simulink model "test_Cart_ver6"  (R2018a)
settings: Solver=VariableStepAuto  StartTime=0.0  StopTime=inf  RelTol=1e-3
undefined symbols (not defined in the file): first, serial, termDistance
libraries: instrumentlib x3, sldrtlib x1, simulink x1
settings Model: Creator=tomato  LastModifiedBy=tomatoPC
settings CodeAppCC: StateflowObjectComments=on

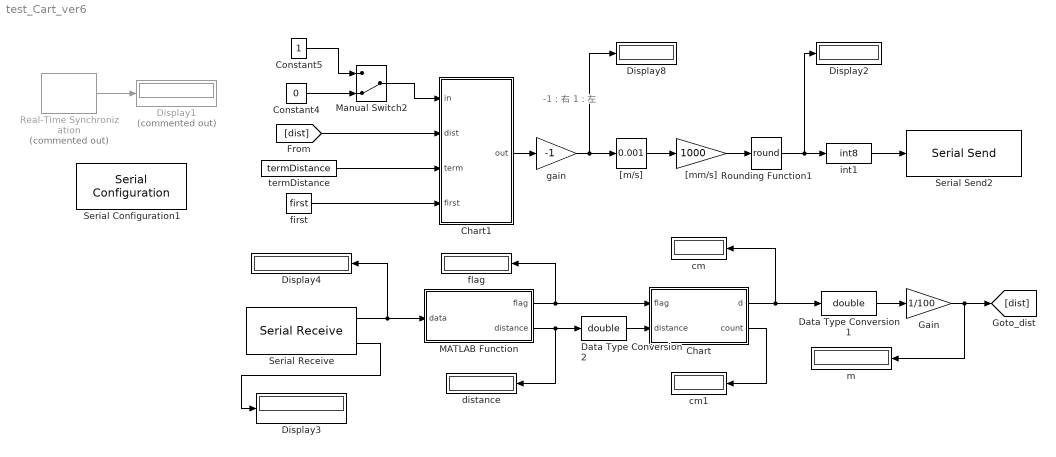
== system test_Cart_ver6 ==
  note: -1 : 右
      | 1 : 左
  Chart : Stateflow chart  TreatAsAtomicUnit=on
  Chart1 : Stateflow chart  TreatAsAtomicUnit=on
  Constant4 : Constant  Value=0  SampleTime=1
  Constant5 : Constant  SampleTime=1
  Data Type Conversion1 : DataTypeConversion  OutDataTypeStr=double
  Data Type Conversion2 : DataTypeConversion  OutDataTypeStr=double
  Display1 : Display  Commented=on
  Display{2..4,8} (4 alike) : Display
  Gain : Gain  Gain=1/100
  MATLAB Function : MATLAB Function  TreatAsAtomicUnit=on
  Manual Switch2 : ManualSwitch  CurrentSetting=0
  Real-Time Synchronization : sldrtlib/Real-Time Synchronization  Commented=on  SampleTime=1  MaxMissedTicks=inf  ShowMissedTicks=on  YieldWhenWaiting=off
  Rounding Function1 : Rounding  Operator=round
  Serial Configuration1 : instrumentlib/Serial Configuration  Priority=-200000  ComPortMenu=<Please select a port...>  ComPort=COM8  ObjConstructor=serial('COM8');  BaudRate=115200  DataBits=8  Parity=none  StopBits=1  FlowControl=none  Timeout=10  ByteOrder=LittleEndian
  Serial Receive : instrumentlib/Serial Receive  ComPortMenu=<Please select a port...>  ComPort=COM8  ObjConstructor=serial('COM8');  Terminator=<none>  DataSize=1  DataType=uint8  EnableBlockingMode=off  ActionDataUnavailable=Output last received value  CustomValue=0  SampleTime=0.01
  Serial Send2 : instrumentlib/Serial Send  ComPortMenu=<Please select a port...>  ComPort=COM8  ObjConstructor=serial('COM8');  Terminator=<none>  EnableBlockingMode=on
  "[m/s]" : simulink/Math Operations/Slider Gain  gain=0.001  low=-0.128  high=0.127
  "[mm/s]" : Gain  Gain=1000
  cm : Display
  cm1 : Display
  distance : Display
  first : Constant  Value=first  SampleTime=1
  flag : Display
  gain : Gain  Gain=-1
  int1 : DataTypeConversion  OutDataTypeStr=int8
  m : Display
  termDistance : Constant  Value=termDistance  SampleTime=1
  wires:
  gain/1 -> "[m/s]"/1, Display8/1
  "[m/s]"/1 -> "[mm/s]"/1
  int1/1 -> Serial Send2/1
  Serial Receive/2 -> Display3/1
  Chart1/1(out) -> gain/1
  "[mm/s]"/1 -> Rounding Function1/1
  termDistance/1 -> Chart1/3(term)
  Manual Switch2/1 -> Chart1/1(in)
  Data Type Conversion1/1 -> Gain/1
  Constant5/1 -> Manual Switch2/1
  Constant4/1 -> Manual Switch2/2
  first/1 -> Chart1/4(first)
  Gain/1 -> m/1, [dist]
  Serial Receive/1 -> MATLAB Function/1(data), Display4/1
  Rounding Function1/1 -> Display2/1, int1/1
  Real-Time Synchronization/1 -> Display1/1
  MATLAB Function/2(distance) -> distance/1, Data Type Conversion2/1
  MATLAB Function/1(flag) -> flag/1, Chart/1(flag)
  [dist] -> Chart1/2(dist)
  Chart/1(d) -> cm/1, Data Type Conversion1/1
  Data Type Conversion2/1 -> Chart/2(distance)
  Chart/2(count) -> cm1/1

== stateflow chart test_Cart_ver6/Chart1 ==
  state CartWait/
    entry:out=0;
  state CartGo1/
    entry:out=0;
  state CartGo3/
    entry:
    flag=flag*-1;
    t=t+term;
  state CartGo2/
    entry:out=flag;
  (default) -> CartWait : {
      | out = 0;
      | flag=1;
      | t=term+first;
      | }
  CartGo2 -> CartWait [order 1] : [in == 0]
  CartWait -> CartGo1 : [in == 1]
  CartGo1 -> CartGo3 [order 2] : [dist >= t ]
  CartGo1 -> CartGo2 [order 1] : [dist < t ]
  CartGo2 -> CartGo3 [order 2] : [dist >= t ]
  CartGo3 -> CartGo2
  data: in input; out output; dist input; term input; flag local; t local; first input double size=1

== stateflow chart test_Cart_ver6/Chart ==
  state mode0/
  state mode1/
    entry:
    count = count;
    d = (count * 127) + distance;
    during:
    d = distance + count * 126;
    count = count;
  (default) -> mode0 : {
      | d = 0;
      | count = 0;
      | }
  mode0 -> mode1
  mode1 -> mode1 : [flag == 1]
      | {
      | count = count + 1;
      | }
  data: flag input; distance input; d output double; count output

== matlab function test_Cart_ver6/MATLAB Function ==
  data: flag output; data input; distance output
function [flag,distance] = fcn(data)

% 入力(data)を右に7bitシフトして、上位1bitを取り出す
flag = uint8(bitshift(data,-7));

% 入力(data)と127(01111111)のAND演算をして、下位7bitを取り出す
distance = uint8( bitand(data, 127));
